simulink model "H2_Z"  (R2020b)
settings: Solver=VariableStepAuto  StartTime=0.0  StopTime=10.0  RelTol=1e-3
settings Model: Creator=intel  LastModifiedBy=intel
settings DataIOCC: SaveOutput=off  SaveTime=off

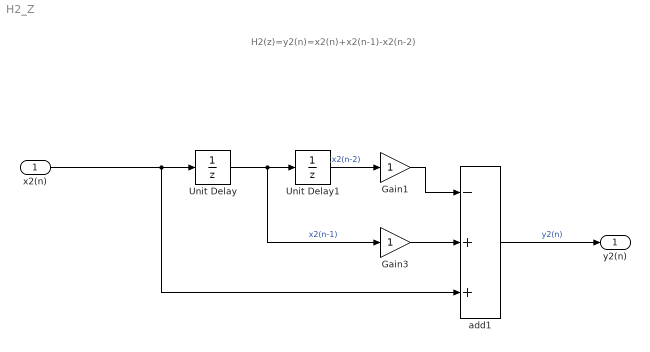
== system H2_Z ==
  note: H2(z)=y2(n)=x2(n)+x2(n-1)-x2(n-2)
  x2(n) : Inport  OutDataTypeStr=double  PortDimensions=1  SampleTime=0
  Gain1 : Gain
  Gain3 : Gain
  Unit Delay : UnitDelay  SampleTime=-1  HasFrameUpgradeWarning=on
  Unit Delay1 : UnitDelay  SampleTime=-1  HasFrameUpgradeWarning=on
  add1 : Sum  Inputs=-++
  y2(n) : Outport  OutDataTypeStr=double  PortDimensions=1  SampleTime=0
  wires:
  Unit Delay/1 -> Gain3/1, Unit Delay1/1  "x2(n-1)"
  x2(n)/1 -> add1/3, Unit Delay/1
  Gain3/1 -> add1/2
  Unit Delay1/1 -> Gain1/1  "x2(n-2)"
  Gain1/1 -> add1/1
  add1/1 -> y2(n)/1  "y2(n)"
